simulink model "cppll"  (Simulink 6.6)
settings: Solver=ode45  StartTime=0.0  StopTime=50e-6  RelTol=1e-3
PostLoadFcn:
  | C2 = 17e-12;
  | C1 = 82e-12;
  | R1 = 23e3;
libraries: commsynccomp2 x1
settings Model: Creator=Edwin Pasterkamp  LastModifiedBy=epasterk
settings DebuggingCC: SignalResolutionControl=TryResolveAllWithWarning

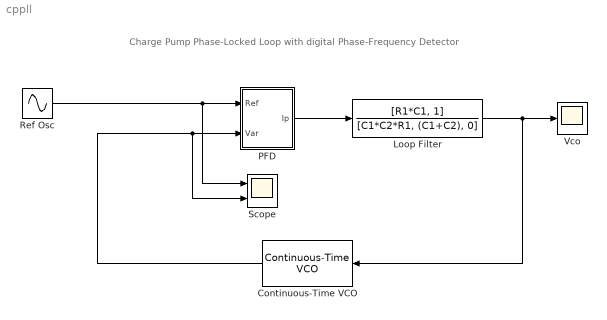
== system cppll ==
  note: Charge Pump Phase-Locked Loop with digital Phase-Frequency Detector
  Continuous-Time VCO : commsynccomp2/Continuous-Time VCO  Orientation=left  SystemSampleTime=-1  Ac=1  Fc=1e6  Kc=3e5 %10e6/32  Ph=-pi/2
  Loop Filter : TransferFcn  Numerator=[R1*C1, 1]  Denominator=[C1*C2*R1, (C1+C2), 0]
  PFD : Subsystem
  Ref Osc : Sin  Frequency=2*pi*1.1e6  SampleTime=0
      settings: AttributesFormatString=%<Frequency> (rad/s)
  Scope : Scope  NumInputPorts=2
      settings: TimeRange=5e-005  YMin=-1.5~-1.5  YMax=1.5~1.5  SampleInput=on  SampleTime=1e-8
  Vco : Scope
      settings: YMin=-30  YMax=30
  wires:
  PFD/1(Ip) -> Loop Filter/1
  Ref Osc/1 -> PFD/1(Ref), Scope/1
  Continuous-Time VCO/1 -> PFD/2(Var), Scope/2
  Loop Filter/1 -> Vco/1, Continuous-Time VCO/1

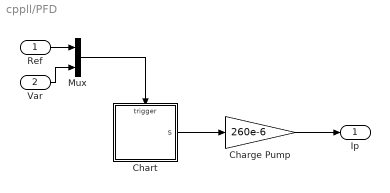
== system cppll/PFD ==
  Ref : Inport
  Var : Inport  Port=2
  Charge Pump : Gain  Gain=260e-6
  Chart : Stateflow chart
  Mux : Mux  Inputs=2
  Ip : Outport
  wires:
  Mux/1 -> Chart/Trigger
  Ref/1 -> Mux/1
  Var/1 -> Mux/2
  Chart/1(s) -> Charge Pump/1
  Charge Pump/1 -> Ip/1

== stateflow chart PFD/Chart ==
  state Ahead
    s = -1;
  state InPhase
    s=0;
  state Behind
    s=1;
  Ahead -> InPhase : ref
  InPhase -> Behind [order 1] : ref
  InPhase -> Ahead [order 2] : var
  Behind -> InPhase : var
  (default) -> InPhase
  data: s output double
  events: ref input RISING_EDGE_EVENT; var input RISING_EDGE_EVENT
